simulink model "EKF"  (R2024b)
settings: Solver=FixedStepAuto  StartTime=0.0  StopTime=10  FixedStep=0.001  RelTol=1e-3
libraries: shared6dof x1, aerolibanim x1, simulink x1, aerolibnav x1
settings Model: Creator=cpero  LastModifiedBy=cpero

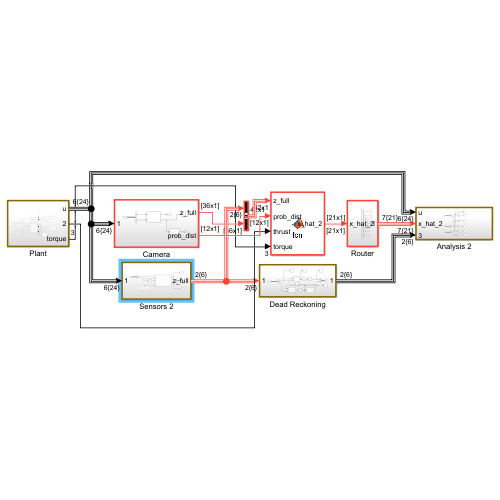
[thumbnail: Simulink's stored preview of the top-level diagram]
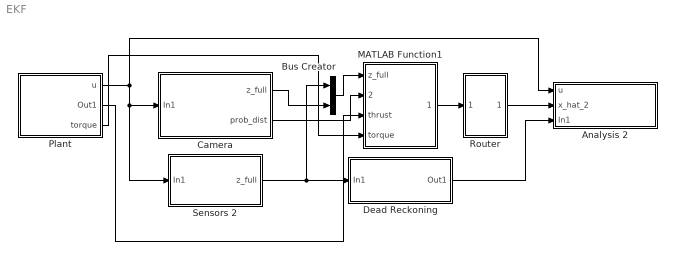
== system EKF ==
  Analysis 2 : Subsystem
  Bus Creator : BusCreator  Inputs=2
  Camera : Subsystem
  Dead Reckoning : Subsystem
  MATLAB Function1 : MATLAB Function  TreatAsAtomicUnit=on
  Plant : Subsystem
  Router : Subsystem
  Sensors 2 : Subsystem
  wires:
  Plant/1(u) -> Camera/1(In1), Sensors 2/1(In1), Analysis 2/1(u)
  Sensors 2/1(z_full) -> Bus Creator/1, Dead Reckoning/1(In1)
  Dead Reckoning/1(Out1) -> Analysis 2/3(In1)
  Router/1(Out1) -> Analysis 2/2(x_hat_2)
  MATLAB Function1/1(x_hat_2) -> Router/1(x_hat_2)
  Bus Creator/1 -> MATLAB Function1/1(z_full)
  Camera/1(z_full) -> Bus Creator/2
  Plant/2(Out1) -> MATLAB Function1/3(thrust)
  Camera/2(prob_dist) -> MATLAB Function1/2(prob_dist)
  Plant/3(torque) -> MATLAB Function1/4(torque)

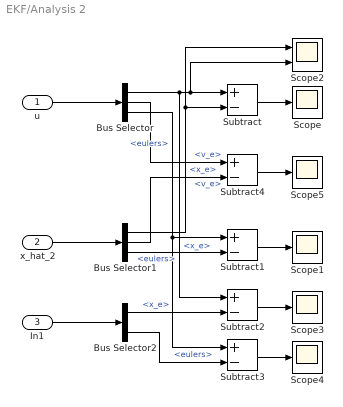
== system EKF/Analysis 2 ==
  u : Inport
  x_hat_2 : Inport  Port=2
  In1 : Inport  Port=3
  Bus Selector : BusSelector  OutputSignals=x_e,v_e,eulers
  Bus Selector1 : BusSelector  OutputSignals=x_e,v_e,eulers
  Bus Selector2 : BusSelector  OutputSignals=x_e,eulers
  Scope{,1,3..5} (5 alike) : Scope
  Scope2 : Scope  NumInputPorts=2
  Subtract{,1..4} (5 alike) : Sum  Inputs=+-
  wires:
  u/1 -> Bus Selector/1
  In1/1 -> Bus Selector2/1
  x_hat_2/1 -> Bus Selector1/1
  Bus Selector/1 -> Subtract2/1, Scope2/2, Subtract/1  "<x_e>"
  Bus Selector1/1 -> Scope2/1, Subtract/2  "<x_e>"
  Subtract/1 -> Scope/1
  Subtract1/1 -> Scope1/1
  Bus Selector/3 -> Subtract3/1, Subtract1/1  "<eulers>"
  Bus Selector1/3 -> Subtract1/2  "<eulers>"
  Subtract2/1 -> Scope3/1
  Bus Selector2/2 -> Subtract3/2  "<eulers>"
  Bus Selector2/1 -> Subtract2/2  "<x_e>"
  Subtract3/1 -> Scope4/1
  Subtract4/1 -> Scope5/1
  Bus Selector/2 -> Subtract4/1  "<v_e>"
  Bus Selector1/2 -> Subtract4/2  "<v_e>"

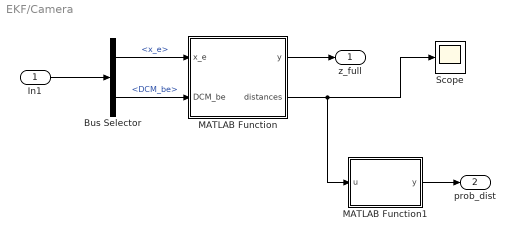
== system EKF/Camera ==
  In1 : Inport
  Bus Selector : BusSelector  OutputSignals=x_e,DCM_be
  MATLAB Function : MATLAB Function  TreatAsAtomicUnit=on
  MATLAB Function1 : MATLAB Function  TreatAsAtomicUnit=on
  Scope : Scope
  z_full : Outport
  prob_dist : Outport  Port=2
  wires:
  In1/1 -> Bus Selector/1
  Bus Selector/1 -> MATLAB Function/1(x_e)  "<x_e>"
  Bus Selector/2 -> MATLAB Function/2(DCM_be)  "<DCM_be>"
  MATLAB Function/1(y) -> z_full/1
  MATLAB Function/2(distances) -> MATLAB Function1/1(u), Scope/1
  MATLAB Function1/1(y) -> prob_dist/1

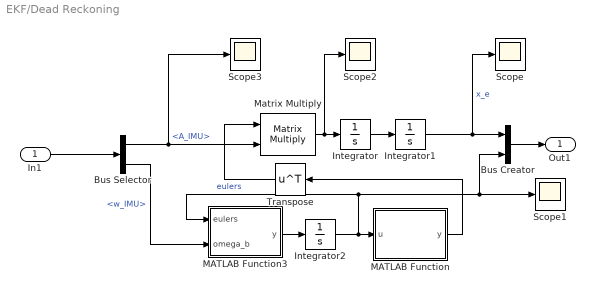
== system EKF/Dead Reckoning ==
  In1 : Inport
  Bus Creator : BusCreator  Inputs=2
  Bus Selector : BusSelector  OutputSignals=A_IMU,w_IMU
  Integrator : Integrator  InitialCondition=[0 0 1]
  Integrator1 : Integrator  InitialCondition=[0 0 1]
  Integrator2 : Integrator  InitialCondition=[0;0;0];
  MATLAB Function : MATLAB Function  TreatAsAtomicUnit=on
  MATLAB Function3 : MATLAB Function  TreatAsAtomicUnit=on
  Matrix Multiply : Product  Multiplication=Matrix(*)
  Scope{,1..3} (4 alike) : Scope
  Transpose : Math  Operator=transpose
  Out1 : Outport
  wires:
  Matrix Multiply/1 -> Scope2/1, Integrator/1
  Integrator/1 -> Integrator1/1
  In1/1 -> Bus Selector/1
  MATLAB Function3/1(y) -> Integrator2/1
  Integrator2/1 -> MATLAB Function/1(u), MATLAB Function3/1(eulers), Bus Creator/2, Scope1/1  "eulers"
  Integrator1/1 -> Scope/1, Bus Creator/1  "x_e"
  Bus Creator/1 -> Out1/1
  MATLAB Function/1(y) -> Transpose/1
  Transpose/1 -> Matrix Multiply/1
  Bus Selector/1 -> Scope3/1, Matrix Multiply/2  "<A_IMU>"
  Bus Selector/2 -> MATLAB Function3/2(omega_b)  "<w_IMU>"

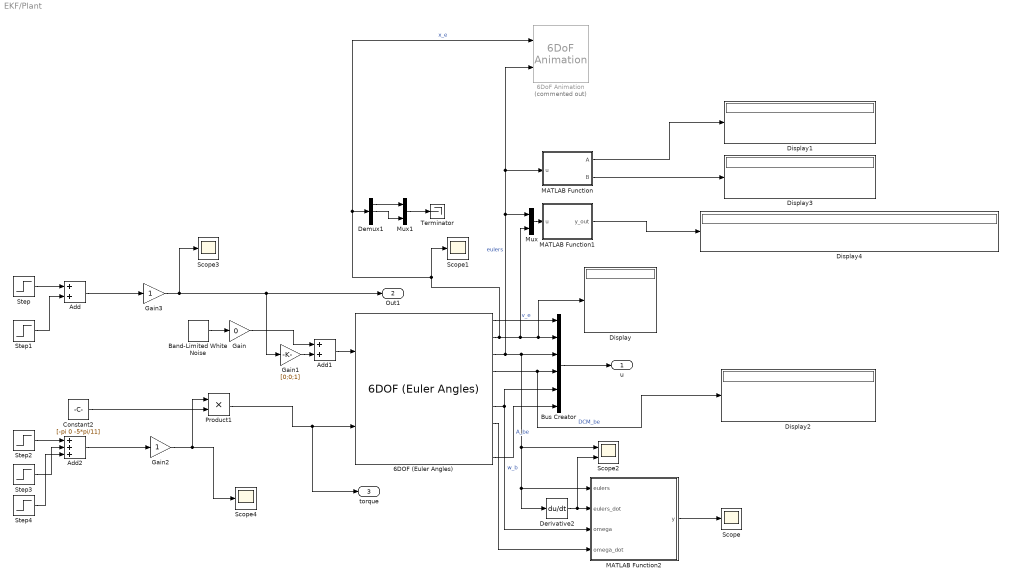
== system EKF/Plant ==
  6DOF (Euler Angles) : shared6dof/6DOF (Euler Angles)  units=Metric (MKS)  mtype=Fixed  rep=Euler Angles  xme_0=[0 0 1]  Vm_0=[0 0 1]  eul_0=[0 0 0]  pm_0=[0 0 0]  mass_0=1.0  mass_e=0.5  mass_f=2.0  inertia=eye(3)  inertia_e=eye(3)  inertia_f=2*eye(3)  k_quat=1.0  vre_flag=on  abi_flag=on  aMode=0  xme_statename=''  Vm_statename=''  eul_statename=''  quat_statename=''  pm_statename=''  mass_statename=''
  6DoF Animation : aerolibanim/6DoF Animation  Commented=on  u1=[-50 50 -50 50 0 50]  u2=0.1  u3=1.0  u4=[0 0 0]  u5=Cockpit  u6=[20 5 -31]  u7=10  u8=on
  Add : Sum
  Add1 : Sum
  Add2 : Sum  Inputs=+++
  Band-Limited White Noise : simulink/Sources/Band-Limited White Noise  Cov=[1e-5 1e-5 1e-5]  Ts=1e-3  seed=[76 34 60]
  Bus Creator : BusCreator  Inputs=6
  Constant2 : Constant  Value=[-pi 0 -5*pi/11]
  Demux1 : Demux  Outputs=3
  Derivative2 : Derivative
  Display{,1..4} (5 alike) : Display
  Gain : Gain  Gain=0
  Gain1 : Gain  Gain=[0;0;1]
  Gain2 : Gain
  Gain3 : Gain
  MATLAB Function : MATLAB Function  TreatAsAtomicUnit=on
  MATLAB Function1 : MATLAB Function  TreatAsAtomicUnit=on
  MATLAB Function2 : MATLAB Function  TreatAsAtomicUnit=on
  Mux : Mux  Inputs=2
  Mux1 : Mux  Inputs=2
  Product1 : Product
  Scope{,1,3..4} (4 alike) : Scope
  Scope2 : Scope  NumInputPorts=2
  Step : Step  SampleTime=0
  Step1 : Step  Time=2  After=-1  SampleTime=0
  Step2 : Step  Time=5  SampleTime=0
  Step3 : Step  Time=6  After=-2  SampleTime=0
  Step4 : Step  Time=7  SampleTime=0
  Terminator : Terminator
  u : Outport
  Out1 : Outport  Port=2
  torque : Outport  Port=3
  wires:
  6DOF (Euler Angles)/2 -> 6DoF Animation/1, Demux1/1, Scope1/1, Mux/2, Display/1, Bus Creator/2  "x_e"
  Bus Creator/1 -> u/1
  6DOF (Euler Angles)/4 -> Display2/1, Bus Creator/4  "DCM_be"
  6DOF (Euler Angles)/3 -> Mux/1, 6DoF Animation/2, MATLAB Function/1(u), MATLAB Function2/1(eulers), Derivative2/1, Scope2/1, Bus Creator/3  "eulers"
  6DOF (Euler Angles)/1 -> Bus Creator/1  "v_e"
  6DOF (Euler Angles)/9 -> Bus Creator/6  "A_be"
  6DOF (Euler Angles)/6 -> MATLAB Function2/3(omega), Bus Creator/5  "w_b"
  MATLAB Function/1(A) -> Display1/1
  MATLAB Function/2(B) -> Display3/1
  MATLAB Function1/1(y_out) -> Display4/1
  Mux/1 -> MATLAB Function1/1(u)
  6DOF (Euler Angles)/7 -> MATLAB Function2/4(omega_dot)
  Derivative2/1 -> Scope2/2, MATLAB Function2/2(eulers_dot)
  MATLAB Function2/1(y) -> Scope/1
  Constant2/1 -> Product1/2
  Demux1/2 -> Mux1/2
  Demux1/1 -> Mux1/1
  Mux1/1 -> Terminator/1
  Band-Limited White Noise/1 -> Gain/1
  Add1/1 -> 6DOF (Euler Angles)/1
  Gain/1 -> Add1/1
  Gain1/1 -> Add1/2
  Gain3/1 -> Scope3/1, Out1/1, Gain1/1
  Add2/1 -> Gain2/1
  Gain2/1 -> Scope4/1, Product1/1
  Step/1 -> Add/1
  Step1/1 -> Add/2
  Add/1 -> Gain3/1
  Step3/1 -> Add2/2
  Step2/1 -> Add2/1
  Step4/1 -> Add2/3
  Product1/1 -> torque/1, 6DOF (Euler Angles)/2

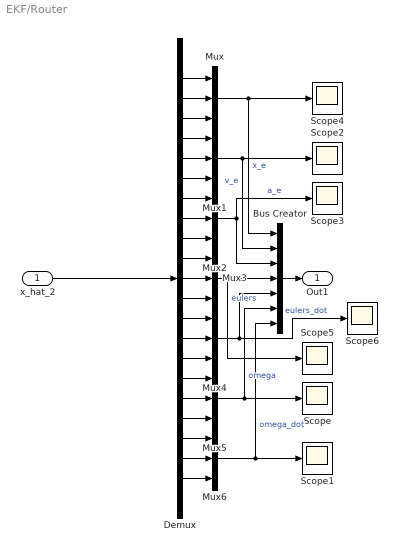
== system EKF/Router ==
  x_hat_2 : Inport
  Bus Creator : BusCreator  Inputs=7
  Demux : Demux  Outputs=21
  Mux{,1..6} (7 alike) : Mux  Inputs=3
  Scope{,1..6} (7 alike) : Scope
  Out1 : Outport
  wires:
  Demux/6 -> Mux1/3
  Mux2/1 -> Scope3/1, Bus Creator/3  "a_e"
  Demux/1 -> Mux/1
  Demux/15 -> Mux4/3
  Demux/18 -> Mux5/3
  Demux/12 -> Mux3/3
  Demux/13 -> Mux4/1
  Mux4/1 -> Scope6/1, Bus Creator/5  "eulers_dot"
  Demux/11 -> Mux3/2
  Mux5/1 -> Bus Creator/6, Scope/1  "omega"
  Demux/14 -> Mux4/2
  Demux/10 -> Mux3/1
  Mux1/1 -> Scope2/1, Bus Creator/2  "v_e"
  Demux/7 -> Mux2/1
  Demux/17 -> Mux5/2
  Demux/2 -> Mux/2
  Demux/5 -> Mux1/2
  Demux/4 -> Mux1/1
  Mux3/1 -> Scope5/1, Bus Creator/4  "eulers"
  Demux/3 -> Mux/3
  Demux/8 -> Mux2/2
  Demux/9 -> Mux2/3
  Demux/19 -> Mux6/1
  Mux/1 -> Scope4/1, Bus Creator/1  "x_e"
  Demux/16 -> Mux5/1
  Demux/20 -> Mux6/2
  Demux/21 -> Mux6/3
  Mux6/1 -> Bus Creator/7, Scope1/1  "omega_dot"
  x_hat_2/1 -> Demux/1
  Bus Creator/1 -> Out1/1

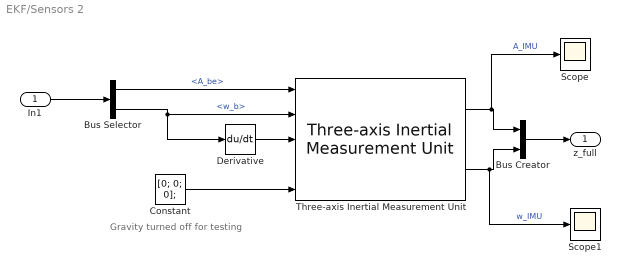
== system EKF/Sensors 2 ==
  note: Gravity turned off for testing
  In1 : Inport
  Bus Creator : BusCreator  Inputs=2
  Bus Selector : BusSelector  OutputSignals=A_be,w_b
  Constant : Constant  Value=[0; 0; 0];
  Derivative : Derivative
  Scope : Scope
  Scope1 : Scope
  Three-axis Inertial Measurement Unit : aerolibnav/Three-axis Inertial Measurement Unit  units=Metric (MKS)  imu=[0 0 0]  i_Ts=1e-3  dtype_a=off  w_a=190  z_a=0.707  a_sf_cc=[1 0 0; 0 1 0; 0 0 1]  a_bias=[0.02 -0.01 0.03]  a_sat="[-inf  -inf  -inf  inf inf inf]"  dtype_g=off  w_g=190  z_g=0.707  g_sf_cc=[1 0 0; 0 1 0; 0 0 1]  g_bias=[0.01 -0.02 0.03]  g_sens=[0 0 0]  g_sat="[-inf  -inf  -inf  inf inf inf]"  i_rand=on  i_seeds=[23093 23094 23095 23096 23097 23098]  i_pow=[1e-4 1e-4 1e-4 1e-6 1e-6 1e-6]
  z_full : Outport
  wires:
  In1/1 -> Bus Selector/1
  Bus Selector/1 -> Three-axis Inertial Measurement Unit/1  "<A_be>"
  Bus Selector/2 -> Derivative/1, Three-axis Inertial Measurement Unit/2  "<w_b>"
  Derivative/1 -> Three-axis Inertial Measurement Unit/3
  Constant/1 -> Three-axis Inertial Measurement Unit/5
  Three-axis Inertial Measurement Unit/1 -> Scope/1, Bus Creator/1  "A_IMU"
  Three-axis Inertial Measurement Unit/2 -> Scope1/1, Bus Creator/2  "w_IMU"
  Bus Creator/1 -> z_full/1

== matlab function EKF/Dead Reckoning/MATLAB Function3 ==
  data: eulers input; y output; omega_b input
function y = fcn(eulers, omega_b)

phi = eulers(1);
theta = eulers(2);
psi = eulers(3);

L = [1 sin(phi)*tan(theta) cos(phi)*tan(theta);
     0 cos(phi) -sin(phi);
     0 sin(phi)*sec(theta) cos(phi)*sec(theta)];

y = L*omega_b;

== matlab function EKF/Dead Reckoning/MATLAB Function ==
  data: u input; y output
function y = fcn(u)

y = angle2dcm(u(3),u(2),u(1));

phi = u(1);
theta = u(2);
psi = u(3);

B = [cos(psi)*cos(theta), cos(theta)*sin(psi), -sin(theta);
     cos(psi)*sin(theta)*sin(phi)-cos(phi)*sin(psi), cos(psi)*cos(phi)+sin(psi)*sin(theta)*sin(phi), cos(theta)*sin(phi);
     sin(psi)*sin(phi)+cos(psi)*cos(phi)*sin(theta), cos(phi)*sin(psi)*sin(theta)-cos(psi)*sin(phi), cos(theta)*cos(phi)];

== matlab function EKF/Plant/MATLAB Function ==
  data: u input; A output; B output
function [A, B] = fcn(u)

%phi
phi = u(1);
c = u(1);

theta = u(2);
b = u(2);

psi = u(3);
a = u(3);

%https://en.wikipedia.org/wiki/Euler_angles
%Transpose to go from DCM_eb to DCM_be
A = [cos(a)*cos(b), cos(a)*sin(b)*sin(c)-cos(c)*sin(a), sin(a)*sin(c)+cos(a)*cos(c)*sin(b);
     cos(b)*sin(a), cos(a)*cos(c)+sin(a)*sin(b)*sin(c), cos(c)*sin(a)*sin(b)-cos(a)*sin(c);
     -sin(b), cos(b)*sin(c), cos(b)*cos(c)]';

B = [cos(psi)*cos(theta), cos(theta)*sin(psi), -sin(theta);
     cos(psi)*sin(theta)*sin(phi)-cos(phi)*sin(psi), cos(psi)*cos(phi)+sin(psi)*sin(theta)*sin(phi), cos(theta)*sin(phi);
     sin(psi)*sin(phi)+cos(psi)*cos(phi)*sin(theta), cos(phi)*sin(psi)*sin(theta)-cos(psi)*sin(phi), cos(theta)*cos(phi)];

== matlab function EKF/Plant/MATLAB Function1 ==
  data: u input; y_out output
function y_out = fcn(u)

phi=u(1);
theta=u(2);
psi=u(3);
x=u(4);
y=u(5);
z=u(6);
a=-50;
b=120;
c=1;

y_out = reshape([0.0,1.0./sqrt((a-x).^2+(b-y).^2+(c-z).^2).*((sin(phi).*sin(psi)+cos(phi).*cos(psi).*sin(theta)).*(a-x)-(cos(psi).*sin(phi)-cos(phi).*sin(psi).*sin(theta)).*(b-y)+cos(phi).*cos(theta).*(c-z)),-1.0./sqrt((a-x).^2+(b-y).^2+(c-z).^2).*(-(cos(phi).*sin(psi)-cos(psi).*sin(phi).*sin(theta)).*(a-x)+(cos(phi).*cos(psi)+sin(phi).*sin(psi).*sin(theta)).*(b-y)+cos(theta).*sin(phi).*(c-z)),-1.0./sqrt((a-x).^2+(b-y).^2+(c-z).^2).*(cos(theta).*(c-z)+cos(psi).*sin(theta).*(a-x)+sin(psi).*sin(theta).*(b-y)),(-sin(phi).*sin(theta).*(c-z)+cos(psi).*cos(theta).*sin(phi).*(a-x)+cos(theta).*sin(phi).*sin(psi).*(b-y)).*1.0./sqrt((a-x).^2+(b-y).^2+(c-z).^2),(-cos(phi).*sin(theta).*(c-z)+cos(phi).*cos(psi).*cos(theta).*(a-x)+cos(phi).*cos(theta).*sin(psi).*(b-y)).*1.0./sqrt((a-x).^2+(b-y).^2+(c-z).^2),(cos(psi).*cos(theta).*(b-y)-cos(theta).*sin(psi).*(a-x)).*1.0./sqrt((a-x).^2+(b-y).^2+(c-z).^2),-((cos(phi).*cos(psi)+sin(phi).*sin(psi).*sin(theta)).*(a-x)+(cos(phi).*sin(psi)-cos(psi).*sin(phi).*sin(theta)).*(b-y)).*1.0./sqrt((a-x).^2+(b-y).^2+(c-z).^2),((cos(psi).*sin(phi)-cos(phi).*sin(psi).*sin(theta)).*(a-x)+(sin(phi).*sin(psi)+cos(phi).*cos(psi).*sin(theta)).*(b-y)).*1.0./sqrt((a-x).^2+(b-y).^2+(c-z).^2),((a.*2.0-x.*2.0).*1.0./((a-x).^2+(b-y).^2+(c-z).^2).^(3.0./2.0).*(-sin(theta).*(c-z)+cos(psi).*cos(theta).*(a-x)+cos(theta).*sin(psi).*(b-y)))./2.0-cos(psi).*cos(theta).*1.0./sqrt((a-x).^2+(b-y).^2+(c-z).^2),(cos(phi).*sin(psi)-cos(psi).*sin(phi).*sin(theta)).*1.0./sqrt((a-x).^2+(b-y).^2+(c-z).^2)+((a.*2.0-x.*2.0).*1.0./((a-x).^2+(b-y).^2+(c-z).^2).^(3.0./2.0).*(-(cos(phi).*sin(psi)-cos(psi).*sin(phi).*sin(theta)).*(a-x)+(cos(phi).*cos(psi)+sin(phi).*sin(psi).*sin(theta)).*(b-y)+cos(theta).*sin(phi).*(c-z)))./2.0,-(sin(phi).*sin(psi)+cos(phi).*cos(psi).*sin(theta)).*1.0./sqrt((a-x).^2+(b-y).^2+(c-z).^2)+((a.*2.0-x.*2.0).*1.0./((a-x).^2+(b-y).^2+(c-z).^2).^(3.0./2.0).*((sin(phi).*sin(psi)+cos(phi).*cos(psi).*sin(theta)).*(a-x)-(cos(psi).*sin(phi)-cos(phi).*sin(psi).*sin(theta)).*(b-y)+cos(phi).*cos(theta).*(c-z)))./2.0,((b.*2.0-y.*2.0).*1.0./((a-x).^2+(b-y).^2+(c-z).^2).^(3.0./2.0).*(-sin(theta).*(c-z)+cos(psi).*cos(theta).*(a-x)+cos(theta).*sin(psi).*(b-y)))./2.0-cos(theta).*sin(psi).*1.0./sqrt((a-x).^2+(b-y).^2+(c-z).^2),-(cos(phi).*cos(psi)+sin(phi).*sin(psi).*sin(theta)).*1.0./sqrt((a-x).^2+(b-y).^2+(c-z).^2)+((b.*2.0-y.*2.0).*1.0./((a-x).^2+(b-y).^2+(c-z).^2).^(3.0./2.0).*(-(cos(phi).*sin(psi)-cos(psi).*sin(phi).*sin(theta)).*(a-x)+(cos(phi).*cos(psi)+sin(phi).*sin(psi).*sin(theta)).*(b-y)+cos(theta).*sin(phi).*(c-z)))./2.0,(cos(psi).*sin(phi)-cos(phi).*sin(psi).*sin(theta)).*1.0./sqrt((a-x).^2+(b-y).^2+(c-z).^2)+((b.*2.0-y.*2.0).*1.0./((a-x).^2+(b-y).^2+(c-z).^2).^(3.0./2.0).*((sin(phi).*sin(psi)+cos(phi).*cos(psi).*sin(theta)).*(a-x)-(cos(psi).*sin(phi)-cos(phi).*sin(psi).*sin(theta)).*(b-y)+cos(phi).*cos(theta).*(c-z)))./2.0,sin(theta).*1.0./sqrt((a-x).^2+(b-y).^2+(c-z).^2)+((c.*2.0-z.*2.0).*1.0./((a-x).^2+(b-y).^2+(c-z).^2).^(3.0./2.0).*(-sin(theta).*(c-z)+cos(psi).*cos(theta).*(a-x)+cos(theta).*sin(psi).*(b-y)))./2.0,-cos(theta).*sin(phi).*1.0./sqrt((a-x).^2+(b-y).^2+(c-z).^2)+((c.*2.0-z.*2.0).*1.0./((a-x).^2+(b-y).^2+(c-z).^2).^(3.0./2.0).*(-(cos(phi).*sin(psi)-cos(psi).*sin(phi).*sin(theta)).*(a-x)+(cos(phi).*cos(psi)+sin(phi).*sin(psi).*sin(theta)).*(b-y)+cos(theta).*sin(phi).*(c-z)))./2.0,-cos(phi).*cos(theta).*1.0./sqrt((a-x).^2+(b-y).^2+(c-z).^2)+((c.*2.0-z.*2.0).*1.0./((a-x).^2+(b-y).^2+(c-z).^2).^(3.0./2.0).*((sin(phi).*sin(psi)+cos(phi).*cos(psi).*sin(theta)).*(a-x)-(cos(psi).*sin(phi)-cos(phi).*sin(psi).*sin(theta)).*(b-y)+cos(phi).*cos(theta).*(c-z)))./2.0],[3,6]);

== matlab function EKF/Plant/MATLAB Function2 ==
  data: eulers input; eulers_dot input; omega input; y output; omega_dot input
function y = fcn(eulers, eulers_dot, omega, omega_dot)

phi = eulers(1);
theta = eulers(2);
psi = eulers(3);
phi_dot = eulers_dot(1);
theta_dot = eulers_dot(2);
psi_dot = eulers_dot(3);

L = [1 sin(phi)*tan(theta) cos(phi)*tan(theta);
     0 cos(phi) -sin(phi);
     0 sin(phi)*sec(theta) cos(phi)*sec(theta)];

L_prime = [0, sin(phi)*(sec(theta)^2)*theta_dot + tan(theta)*cos(phi)*phi_dot, cos(phi)*(sec(theta)^2)*theta_dot - tan(theta)*sin(phi)*phi_dot;
           0, -sin(phi)*phi_dot, -cos(phi)*phi_dot;
           0, sin(phi)*(tan(theta)*sec(theta))*theta_dot + sec(theta)*cos(phi)*phi_dot, cos(phi)*(tan(theta)*sec(theta))*theta_dot - sec(theta)*sin(phi)*phi_dot];

y = (L*omega_dot) + (L_prime*omega);

== matlab function EKF/Camera/MATLAB Function ==
  settings: updateMethod=DISCRETE
  data: x_e input; y output; DCM_be input; marker_data parameter; distances output
function [y, distances] = fcn(x_e, DCM_be, marker_data)
N = size(marker_data, 2);

distances = zeros(N,1);
y = zeros(N*3,1);
for i=1:N
    delta = DCM_be*(marker_data(:,i) - x_e);
    rho = delta/(norm(delta));
    distances(i) = norm(delta); 
    y(1+(3*(i-1)):3+(3*(i-1))) = rho + normrnd(0,1e-2,[3,1]);
end

== matlab function EKF/MATLAB Function1 ==
  settings: updateMethod=DISCRETE
  data: z_full input; prob_dist input; x_hat_2 output; marker_data parameter; thrust input; torque input
function x_hat_2  = fcn(z_full, prob_dist, marker_data, thrust, torque)

persistent x_hat_2_prior P_hat_2_prior j

if isempty(x_hat_2_prior)
    x_hat_2_prior = zeros(21,1);
    x_hat_2_prior(1:3) = [0 0 1];
    x_hat_2_prior(4:6) = [0 0 1];
    x_hat_2_prior(7:9) = [0 0 0];
    P_hat_2_prior = kron(diag([1e-4 1e-4 1e-4 1e-4 1e-6 1e-6 1e-6]),eye(3));
    x_hat_2_prior(10:12) = [0 0 0];
    x_hat_2_prior(13:15) = [0 0 0];
    x_hat_2_prior(16:18) = [0 0 0];
    j=0;
end

rho_num = size(marker_data, 2);

accel_vec = ones(1,3);
gyro_vec = ones(1,3);
rho_vec = zeros(1,3*rho_num);

rho_calc_required = false;
if true
    rng(j);
    num_tries=5;
    random_rhos = randi(rho_num,[1,num_tries]);
    for k=1:num_tries
        cdf = cumsum(prob_dist);
        random_value = rand();
        random_rho = find(random_value <= cdf, 1);
        rho_vec(3*(random_rho(1)-1)+1:3*random_rho(1)) = ones(1,3);
    end
    sensor_vec = [accel_vec, gyro_vec, rho_vec];
    rho_calc_required = true;
else
    sensor_vec = [accel_vec, gyro_vec, zeros(1,3*rho_num)];
end

j = j+1;

dt = 1e-3;

Q = kron(diag([0 0 0 0 0 0 0]),eye(3));
rho_R_vec = 1e-2*ones(1,rho_num);
R_full = kron(diag([1e-1 1e-1 rho_R_vec]),eye(3));

[r1, r2, r3] = deal(x_hat_2_prior(1), x_hat_2_prior(2), x_hat_2_prior(3));
[r_dot1, r_dot2, r_dot3] = deal(x_hat_2_prior(4), x_hat_2_prior(5), x_hat_2_prior(6));
[r_dot_dot1, r_dot_dot2, r_dot_dot3] = deal(x_hat_2_prior(7), x_hat_2_prior(8), x_hat_2_prior(9));
[eulers1, eulers2, eulers3] = deal(x_hat_2_prior(10), x_hat_2_prior(11), x_hat_2_prior(12));
[eulers_dot1, eulers_dot2, eulers_dot3] = deal(x_hat_2_prior(13), x_hat_2_prior(14), x_hat_2_prior(15));
[omega1, omega2, omega3] = deal(x_hat_2_prior(16), x_hat_2_prior(17), x_hat_2_prior(18));
[omega_dot1, omega_dot2, omega_dot3] = deal(x_hat_2_prior(19), x_hat_2_prior(20), x_hat_2_prior(21));

torque1 = torque(1); 
torque2 = torque(2);
torque3 = torque(3);
mass = 1;

%Predict
x_hat_1 = [r1+dt.*r_dot1+(dt.^2.*r_dot_dot1)./2.0;r2+dt.*r_dot2+(dt.^2.*r_dot_dot2)./2.0;r3+dt.*r_dot3+(dt.^2.*r_dot_dot3)./2.0;r_dot1+dt.*r_dot_dot1;r_dot2+dt.*r_dot_dot2;r_dot3+dt.*r_dot_dot3;(thrust.*(sin(eulers1).*sin(eulers3)+cos(eulers1).*cos(eulers3).*sin(eulers2)))./mass;-(thrust.*(cos(eulers3).*sin(eulers1)-cos(eulers1).*sin(eulers2).*sin(eulers3)))./mass;(thrust.*cos(eulers1).*cos(eulers2))./mass;eulers1+dt.*eulers_dot1;eulers2+dt.*eulers_dot2;eulers3+dt.*eulers_dot3;eulers_dot1+dt.*(omega_dot1+omega2.*(eulers_dot1.*cos(eulers1).*tan(eulers2)+eulers_dot2.*1.0./cos(eulers2).^2.*sin(eulers1))-omega3.*(eulers_dot1.*sin(eulers1).*tan(eulers2)-eulers_dot2.*cos(eulers1).*1.0./cos(eulers2).^2)+omega_dot3.*cos(eulers1).*tan(eulers2)+omega_dot2.*sin(eulers1).*tan(eulers2));eulers_dot2-dt.*(-omega_dot2.*cos(eulers1)+omega_dot3.*sin(eulers1)+eulers_dot1.*omega2.*sin(eulers1)+eulers_dot1.*omega3.*cos(eulers1));eulers_dot3+dt.*(omega2.*((eulers_dot1.*cos(eulers1))./cos(eulers2)+(eulers_dot2.*sin(eulers1).*tan(eulers2))./cos(eulers2))-omega3.*((eulers_dot1.*sin(eulers1))./cos(eulers2)-(eulers_dot2.*cos(eulers1).*tan(eulers2))./cos(eulers2))+(omega_dot3.*cos(eulers1))./cos(eulers2)+(omega_dot2.*sin(eulers1))./cos(eulers2));omega1+dt.*omega_dot1;omega2+dt.*omega_dot2;omega3+dt.*omega_dot3;torque1;torque2;torque3];
F_jacobian = reshape([1.0,0.0,0.0,0.0,0.0,0.0,0.0,0.0,0.0,0.0,0.0,0.0,0.0,0.0,0.0,0.0,0.0,0.0,0.0,0.0,0.0,0.0,1.0,0.0,0.0,0.0,0.0,0.0,0.0,0.0,0.0,0.0,0.0,0.0,0.0,0.0,0.0,0.0,0.0,0.0,0.0,0.0,0.0,0.0,1.0,0.0,0.0,0.0,0.0,0.0,0.0,0.0,0.0,0.0,0.0,0.0,0.0,0.0,0.0,0.0,0.0,0.0,0.0,dt,0.0,0.0,1.0,0.0,0.0,0.0,0.0,0.0,0.0,0.0,0.0,0.0,0.0,0.0,0.0,0.0,0.0,0.0,0.0,0.0,0.0,dt,0.0,0.0,1.0,0.0,0.0,0.0,0.0,0.0,0.0,0.0,0.0,0.0,0.0,0.0,0.0,0.0,0.0,0.0,0.0,0.0,0.0,dt,0.0,0.0,1.0,0.0,0.0,0.0,0.0,0.0,0.0,0.0,0.0,0.0,0.0,0.0,0.0,0.0,0.0,0.0,dt.^2./2.0,0.0,0.0,dt,0.0,0.0,0.0,0.0,0.0,0.0,0.0,0.0,0.0,0.0,0.0,0.0,0.0,0.0,0.0,0.0,0.0,0.0,dt.^2./2.0,0.0,0.0,dt,0.0,0.0,0.0,0.0,0.0,0.0,0.0,0.0,0.0,0.0,0.0,0.0,0.0,0.0,0.0,0.0,0.0,0.0,dt.^2./2.0,0.0,0.0,dt,0.0,0.0,0.0,0.0,0.0,0.0,0.0,0.0,0.0,0.0,0.0,0.0,0.0,0.0,0.0,0.0,0.0,0.0,0.0,0.0,0.0,(thrust.*(cos(eulers1).*sin(eulers3)-cos(eulers3).*sin(eulers1).*sin(eulers2)))./mass,-(thrust.*(cos(eulers1).*cos(eulers3)+sin(eulers1).*sin(eulers2).*sin(eulers3)))./mass,-(thrust.*cos(eulers2).*sin(eulers1))./mass,1.0,0.0,0.0,-dt.*(omega2.*(eulers_dot1.*sin(eulers1).*tan(eulers2)-eulers_dot2.*cos(eulers1).*1.0./cos(eulers2).^2)+omega3.*(eulers_dot1.*cos(eulers1).*tan(eulers2)+eulers_dot2.*1.0./cos(eulers2).^2.*sin(eulers1))-omega_dot2.*cos(eulers1).*tan(eulers2)+omega_dot3.*sin(eulers1).*tan(eulers2)),-dt.*(omega_dot3.*cos(eulers1)+omega_dot2.*sin(eulers1)-eulers_dot1.*omega3.*sin(eulers1)+eulers_dot1.*omega2.*cos(eulers1)),-dt.*(omega2.*((eulers_dot1.*sin(eulers1))./cos(eulers2)-(eulers_dot2.*cos(eulers1).*tan(eulers2))./cos(eulers2))+omega3.*((eulers_dot1.*cos(eulers1))./cos(eulers2)+(eulers_dot2.*sin(eulers1).*tan(eulers2))./cos(eulers2))-(omega_dot2.*cos(eulers1))./cos(eulers2)+(omega_dot3.*sin(eulers1))./cos(eulers2)),0.0,0.0,0.0,0.0,0.0,0.0,0.0,0.0,0.0,0.0,0.0,0.0,(thrust.*cos(eulers1).*cos(eulers2).*cos(eulers3))./mass,(thrust.*cos(eulers1).*cos(eulers2).*sin(eulers3))./mass,-(thrust.*cos(eulers1).*sin(eulers2))./mass,0.0,1.0,0.0,dt.*(omega2.*(eulers_dot1.*cos(eulers1).*(tan(eulers2).^2+1.0)+eulers_dot2.*1.0./cos(eulers2).^3.*sin(eulers1).*sin(eulers2).*2.0)-omega3.*(eulers_dot1.*sin(eulers1).*(tan(eulers2).^2+1.0)-eulers_dot2.*cos(eulers1).*1.0./cos(eulers2).^3.*sin(eulers2).*2.0)+omega_dot3.*cos(eulers1).*(tan(eulers2).^2+1.0)+omega_dot2.*sin(eulers1).*(tan(eulers2).^2+1.0)),0.0,dt.*(omega3.*((eulers_dot2.*cos(eulers1).*(tan(eulers2).^2+1.0))./cos(eulers2)-eulers_dot1.*1.0./cos(eulers2).^2.*sin(eulers1).*sin(eulers2)+eulers_dot2.*cos(eulers1).*1.0./cos(eulers2).^2.*sin(eulers2).*tan(eulers2))+omega2.*((eulers_dot2.*sin(eulers1).*(tan(eulers2).^2+1.0))./cos(eulers2)+eulers_dot1.*cos(eulers1).*1.0./cos(eulers2).^2.*sin(eulers2)+eulers_dot2.*1.0./cos(eulers2).^2.*sin(eulers1).*sin(eulers2).*tan(eulers2))+omega_dot3.*cos(eulers1).*1.0./cos(eulers2).^2.*sin(eulers2)+omega_dot2.*1.0./cos(eulers2).^2.*sin(eulers1).*sin(eulers2)),0.0,0.0,0.0,0.0,0.0,0.0,0.0,0.0,0.0,0.0,0.0,0.0,(thrust.*(cos(eulers3).*sin(eulers1)-cos(eulers1).*sin(eulers2).*sin(eulers3)))./mass,(thrust.*(sin(eulers1).*sin(eulers3)+cos(eulers1).*cos(eulers3).*sin(eulers2)))./mass,0.0,0.0,0.0,1.0,0.0,0.0,0.0,0.0,0.0,0.0,0.0,0.0,0.0,0.0,0.0,0.0,0.0,0.0,0.0,0.0,0.0,0.0,dt,0.0,0.0,dt.*(omega2.*cos(eulers1).*tan(eulers2)-omega3.*sin(eulers1).*tan(eulers2))+1.0,-dt.*(omega3.*cos(eulers1)+omega2.*sin(eulers1)),dt.*((omega2.*cos(eulers1))./cos(eulers2)-(omega3.*sin(eulers1))./cos(eulers2)),0.0,0.0,0.0,0.0,0.0,0.0,0.0,0.0,0.0,0.0,0.0,0.0,0.0,0.0,0.0,0.0,dt,0.0,dt.*(omega3.*cos(eulers1).*1.0./cos(eulers2).^2+omega2.*1.0./cos(eulers2).^2.*sin(eulers1)),1.0,dt.*((omega3.*cos(eulers1).*tan(eulers2))./cos(eulers2)+(omega2.*sin(eulers1).*tan(eulers2))./cos(eulers2)),0.0,0.0,0.0,0.0,0.0,0.0,0.0,0.0,0.0,0.0,0.0,0.0,0.0,0.0,0.0,0.0,0.0,dt,0.0,0.0,1.0,0.0,0.0,0.0,0.0,0.0,0.0,0.0,0.0,0.0,0.0,0.0,0.0,0.0,0.0,0.0,0.0,0.0,0.0,0.0,0.0,0.0,1.0,0.0,0.0,0.0,0.0,0.0,0.0,0.0,0.0,0.0,0.0,0.0,0.0,0.0,0.0,0.0,0.0,0.0,dt.*(eulers_dot1.*cos(eulers1).*tan(eulers2)+eulers_dot2.*1.0./cos(eulers2).^2.*sin(eulers1)),-dt.*eulers_dot1.*sin(eulers1),dt.*((eulers_dot1.*cos(eulers1))./cos(eulers2)+(eulers_dot2.*sin(eulers1).*tan(eulers2))./cos(eulers2)),0.0,1.0,0.0,0.0,0.0,0.0,0.0,0.0,0.0,0.0,0.0,0.0,0.0,0.0,0.0,0.0,0.0,0.0,-dt.*(eulers_dot1.*sin(eulers1).*tan(eulers2)-eulers_dot2.*cos(eulers1).*1.0./cos(eulers2).^2),-dt.*eulers_dot1.*cos(eulers1),-dt.*((eulers_dot1.*sin(eulers1))./cos(eulers2)-(eulers_dot2.*cos(eulers1).*tan(eulers2))./cos(eulers2)),0.0,0.0,1.0,0.0,0.0,0.0,0.0,0.0,0.0,0.0,0.0,0.0,0.0,0.0,0.0,0.0,0.0,0.0,dt,0.0,0.0,dt,0.0,0.0,0.0,0.0,0.0,0.0,0.0,0.0,0.0,0.0,0.0,0.0,0.0,0.0,0.0,0.0,0.0,dt.*sin(eulers1).*tan(eulers2),dt.*cos(eulers1),(dt.*sin(eulers1))./cos(eulers2),0.0,dt,0.0,0.0,0.0,0.0,0.0,0.0,0.0,0.0,0.0,0.0,0.0,0.0,0.0,0.0,0.0,0.0,dt.*cos(eulers1).*tan(eulers2),-dt.*sin(eulers1),(dt.*cos(eulers1))./cos(eulers2),0.0,0.0,dt,0.0,0.0,0.0],[21,21]);
P_hat_1 = F_jacobian*P_hat_2_prior*F_jacobian' + Q;

%Update
num_states = 21;

rho_prediction = zeros(rho_num*3,1);
H_jacobian_rho = zeros(rho_num*3,21);
if rho_calc_required
    for i=1:rho_num
        marker1 = marker_data(1,i);
        marker2 = marker_data(2,i);
        marker3 = marker_data(3,i);
        rho_prediction(1+(3*(i-1)):3+(3*(i-1))) = [1.0./sqrt((marker1-r1).^2+(marker2-r2).^2+(marker3-r3).^2).*(-sin(eulers2).*(marker3-r3)+cos(eulers2).*cos(eulers3).*(marker1-r1)+cos(eulers2).*sin(eulers3).*(marker2-r2));
            1.0./sqrt((marker1-r1).^2+(marker2-r2).^2+(marker3-r3).^2).*(-(cos(eulers1).*sin(eulers3)-cos(eulers3).*sin(eulers1).*sin(eulers2)).*(marker1-r1)+(cos(eulers1).*cos(eulers3)+sin(eulers1).*sin(eulers2).*sin(eulers3)).*(marker2-r2)+cos(eulers2).*sin(eulers1).*(marker3-r3));
            1.0./sqrt((marker1-r1).^2+(marker2-r2).^2+(marker3-r3).^2).*((sin(eulers1).*sin(eulers3)+cos(eulers1).*cos(eulers3).*sin(eulers2)).*(marker1-r1)-(cos(eulers3).*sin(eulers1)-cos(eulers1).*sin(eulers2).*sin(eulers3)).*(marker2-r2)+cos(eulers1).*cos(eulers2).*(marker3-r3))];
        H_jacobian_rho(1+(3*(i-1)):3+(3*(i-1)),:) = reshape([((marker1.*2.0-r1.*2.0).*1.0./((marker1-r1).^2+(marker2-r2).^2+(marker3-r3).^2).^(3.0./2.0).*(-sin(eulers2).*(marker3-r3)+cos(eulers2).*cos(eulers3).*(marker1-r1)+cos(eulers2).*sin(eulers3).*(marker2-r2)))./2.0-cos(eulers2).*cos(eulers3).*1.0./sqrt((marker1-r1).^2+(marker2-r2).^2+(marker3-r3).^2),(cos(eulers1).*sin(eulers3)-cos(eulers3).*sin(eulers1).*sin(eulers2)).*1.0./sqrt((marker1-r1).^2+(marker2-r2).^2+(marker3-r3).^2)+((marker1.*2.0-r1.*2.0).*1.0./((marker1-r1).^2+(marker2-r2).^2+(marker3-r3).^2).^(3.0./2.0).*(-(cos(eulers1).*sin(eulers3)-cos(eulers3).*sin(eulers1).*sin(eulers2)).*(marker1-r1)+(cos(eulers1).*cos(eulers3)+sin(eulers1).*sin(eulers2).*sin(eulers3)).*(marker2-r2)+cos(eulers2).*sin(eulers1).*(marker3-r3)))./2.0,-(sin(eulers1).*sin(eulers3)+cos(eulers1).*cos(eulers3).*sin(eulers2)).*1.0./sqrt((marker1-r1).^2+(marker2-r2).^2+(marker3-r3).^2)+((marker1.*2.0-r1.*2.0).*1.0./((marker1-r1).^2+(marker2-r2).^2+(marker3-r3).^2).^(3.0./2.0).*((sin(eulers1).*sin(eulers3)+cos(eulers1).*cos(eulers3).*sin(eulers2)).*(marker1-r1)-(cos(eulers3).*sin(eulers1)-cos(eulers1).*sin(eulers2).*sin(eulers3)).*(marker2-r2)+cos(eulers1).*cos(eulers2).*(marker3-r3)))./2.0,((marker2.*2.0-r2.*2.0).*1.0./((marker1-r1).^2+(marker2-r2).^2+(marker3-r3).^2).^(3.0./2.0).*(-sin(eulers2).*(marker3-r3)+cos(eulers2).*cos(eulers3).*(marker1-r1)+cos(eulers2).*sin(eulers3).*(marker2-r2)))./2.0-cos(eulers2).*sin(eulers3).*1.0./sqrt((marker1-r1).^2+(marker2-r2).^2+(marker3-r3).^2),-(cos(eulers1).*cos(eulers3)+sin(eulers1).*sin(eulers2).*sin(eulers3)).*1.0./sqrt((marker1-r1).^2+(marker2-r2).^2+(marker3-r3).^2)+((marker2.*2.0-r2.*2.0).*1.0./((marker1-r1).^2+(marker2-r2).^2+(marker3-r3).^2).^(3.0./2.0).*(-(cos(eulers1).*sin(eulers3)-cos(eulers3).*sin(eulers1).*sin(eulers2)).*(marker1-r1)+(cos(eulers1).*cos(eulers3)+sin(eulers1).*sin(eulers2).*sin(eulers3)).*(marker2-r2)+cos(eulers2).*sin(eulers1).*(marker3-r3)))./2.0,(cos(eulers3).*sin(eulers1)-cos(eulers1).*sin(eulers2).*sin(eulers3)).*1.0./sqrt((marker1-r1).^2+(marker2-r2).^2+(marker3-r3).^2)+((marker2.*2.0-r2.*2.0).*1.0./((marker1-r1).^2+(marker2-r2).^2+(marker3-r3).^2).^(3.0./2.0).*((sin(eulers1).*sin(eulers3)+cos(eulers1).*cos(eulers3).*sin(eulers2)).*(marker1-r1)-(cos(eulers3).*sin(eulers1)-cos(eulers1).*sin(eulers2).*sin(eulers3)).*(marker2-r2)+cos(eulers1).*cos(eulers2).*(marker3-r3)))./2.0,sin(eulers2).*1.0./sqrt((marker1-r1).^2+(marker2-r2).^2+(marker3-r3).^2)+((marker3.*2.0-r3.*2.0).*1.0./((marker1-r1).^2+(marker2-r2).^2+(marker3-r3).^2).^(3.0./2.0).*(-sin(eulers2).*(marker3-r3)+cos(eulers2).*cos(eulers3).*(marker1-r1)+cos(eulers2).*sin(eulers3).*(marker2-r2)))./2.0,((marker3.*2.0-r3.*2.0).*1.0./((marker1-r1).^2+(marker2-r2).^2+(marker3-r3).^2).^(3.0./2.0).*(-(cos(eulers1).*sin(eulers3)-cos(eulers3).*sin(eulers1).*sin(eulers2)).*(marker1-r1)+(cos(eulers1).*cos(eulers3)+sin(eulers1).*sin(eulers2).*sin(eulers3)).*(marker2-r2)+cos(eulers2).*sin(eulers1).*(marker3-r3)))./2.0-cos(eulers2).*sin(eulers1).*1.0./sqrt((marker1-r1).^2+(marker2-r2).^2+(marker3-r3).^2),((marker3.*2.0-r3.*2.0).*1.0./((marker1-r1).^2+(marker2-r2).^2+(marker3-r3).^2).^(3.0./2.0).*((sin(eulers1).*sin(eulers3)+cos(eulers1).*cos(eulers3).*sin(eulers2)).*(marker1-r1)-(cos(eulers3).*sin(eulers1)-cos(eulers1).*sin(eulers2).*sin(eulers3)).*(marker2-r2)+cos(eulers1).*cos(eulers2).*(marker3-r3)))./2.0-cos(eulers1).*cos(eulers2).*1.0./sqrt((marker1-r1).^2+(marker2-r2).^2+(marker3-r3).^2),0.0,0.0,0.0,0.0,0.0,0.0,0.0,0.0,0.0,0.0,0.0,0.0,0.0,0.0,0.0,0.0,0.0,0.0,0.0,1.0./sqrt((marker1-r1).^2+(marker2-r2).^2+(marker3-r3).^2).*((sin(eulers1).*sin(eulers3)+cos(eulers1).*cos(eulers3).*sin(eulers2)).*(marker1-r1)-(cos(eulers3).*sin(eulers1)-cos(eulers1).*sin(eulers2).*sin(eulers3)).*(marker2-r2)+cos(eulers1).*cos(eulers2).*(marker3-r3)),-1.0./sqrt((marker1-r1).^2+(marker2-r2).^2+(marker3-r3).^2).*(-(cos(eulers1).*sin(eulers3)-cos(eulers3).*sin(eulers1).*sin(eulers2)).*(marker1-r1)+(cos(eulers1).*cos(eulers3)+sin(eulers1).*sin(eulers2).*sin(eulers3)).*(marker2-r2)+cos(eulers2).*sin(eulers1).*(marker3-r3)),-1.0./sqrt((marker1-r1).^2+(marker2-r2).^2+(marker3-r3).^2).*(cos(eulers2).*(marker3-r3)+cos(eulers3).*sin(eulers2).*(marker1-r1)+sin(eulers2).*sin(eulers3).*(marker2-r2)),1.0./sqrt((marker1-r1).^2+(marker2-r2).^2+(marker3-r3).^2).*(-sin(eulers1).*sin(eulers2).*(marker3-r3)+cos(eulers2).*cos(eulers3).*sin(eulers1).*(marker1-r1)+cos(eulers2).*sin(eulers1).*sin(eulers3).*(marker2-r2)),1.0./sqrt((marker1-r1).^2+(marker2-r2).^2+(marker3-r3).^2).*(-cos(eulers1).*sin(eulers2).*(marker3-r3)+cos(eulers1).*cos(eulers2).*cos(eulers3).*(marker1-r1)+cos(eulers1).*cos(eulers2).*sin(eulers3).*(marker2-r2)),(cos(eulers2).*cos(eulers3).*(marker2-r2)-cos(eulers2).*sin(eulers3).*(marker1-r1)).*1.0./sqrt((marker1-r1).^2+(marker2-r2).^2+(marker3-r3).^2),-((cos(eulers1).*cos(eulers3)+sin(eulers1).*sin(eulers2).*sin(eulers3)).*(marker1-r1)+(cos(eulers1).*sin(eulers3)-cos(eulers3).*sin(eulers1).*sin(eulers2)).*(marker2-r2)).*1.0./sqrt((marker1-r1).^2+(marker2-r2).^2+(marker3-r3).^2),((cos(eulers3).*sin(eulers1)-cos(eulers1).*sin(eulers2).*sin(eulers3)).*(marker1-r1)+(sin(eulers1).*sin(eulers3)+cos(eulers1).*cos(eulers3).*sin(eulers2)).*(marker2-r2)).*1.0./sqrt((marker1-r1).^2+(marker2-r2).^2+(marker3-r3).^2),0.0,0.0,0.0,0.0,0.0,0.0,0.0,0.0,0.0,0.0,0.0,0.0,0.0,0.0,0.0,0.0,0.0,0.0,0.0,0.0,0.0,0.0,0.0,0.0,0.0,0.0,0.0],[3,21]);
        i = i+1;
    end
end

omega_prediction = [omega1; omega2; omega3];
accel_prediction = [r_dot_dot1; r_dot_dot2; r_dot_dot3];

H_jacobian_accel = reshape([0.0,0.0,0.0,0.0,0.0,0.0,0.0,0.0,0.0,0.0,0.0,0.0,0.0,0.0,0.0,0.0,0.0,0.0,cos(eulers2).*cos(eulers3),-cos(eulers1).*sin(eulers3)+cos(eulers3).*sin(eulers1).*sin(eulers2),sin(eulers1).*sin(eulers3)+cos(eulers1).*cos(eulers3).*sin(eulers2),cos(eulers2).*sin(eulers3),cos(eulers1).*cos(eulers3)+sin(eulers1).*sin(eulers2).*sin(eulers3),-cos(eulers3).*sin(eulers1)+cos(eulers1).*sin(eulers2).*sin(eulers3),-sin(eulers2),cos(eulers2).*sin(eulers1),cos(eulers1).*cos(eulers2),0.0,r_dot_dot1.*(sin(eulers1).*sin(eulers3)+cos(eulers1).*cos(eulers3).*sin(eulers2))-r_dot_dot2.*(cos(eulers3).*sin(eulers1)-cos(eulers1).*sin(eulers2).*sin(eulers3))+r_dot_dot3.*cos(eulers1).*cos(eulers2),r_dot_dot1.*(cos(eulers1).*sin(eulers3)-cos(eulers3).*sin(eulers1).*sin(eulers2))-r_dot_dot2.*(cos(eulers1).*cos(eulers3)+sin(eulers1).*sin(eulers2).*sin(eulers3))-r_dot_dot3.*cos(eulers2).*sin(eulers1),-r_dot_dot3.*cos(eulers2)-r_dot_dot1.*cos(eulers3).*sin(eulers2)-r_dot_dot2.*sin(eulers2).*sin(eulers3),-r_dot_dot3.*sin(eulers1).*sin(eulers2)+r_dot_dot1.*cos(eulers2).*cos(eulers3).*sin(eulers1)+r_dot_dot2.*cos(eulers2).*sin(eulers1).*sin(eulers3),-r_dot_dot3.*cos(eulers1).*sin(eulers2)+r_dot_dot1.*cos(eulers1).*cos(eulers2).*cos(eulers3)+r_dot_dot2.*cos(eulers1).*cos(eulers2).*sin(eulers3),r_dot_dot2.*cos(eulers2).*cos(eulers3)-r_dot_dot1.*cos(eulers2).*sin(eulers3),-r_dot_dot1.*(cos(eulers1).*cos(eulers3)+sin(eulers1).*sin(eulers2).*sin(eulers3))-r_dot_dot2.*(cos(eulers1).*sin(eulers3)-cos(eulers3).*sin(eulers1).*sin(eulers2)),r_dot_dot1.*(cos(eulers3).*sin(eulers1)-cos(eulers1).*sin(eulers2).*sin(eulers3))+r_dot_dot2.*(sin(eulers1).*sin(eulers3)+cos(eulers1).*cos(eulers3).*sin(eulers2)),0.0,0.0,0.0,0.0,0.0,0.0,0.0,0.0,0.0,0.0,0.0,0.0,0.0,0.0,0.0,0.0,0.0,0.0,0.0,0.0,0.0,0.0,0.0,0.0,0.0,0.0,0.0],[3,21]);
H_jacobian_omega = [zeros(3,15),eye(3),zeros(3,3)];

prediction_full = [accel_prediction; omega_prediction; rho_prediction];
H_jacobian_full = [H_jacobian_accel; H_jacobian_omega; H_jacobian_rho];

if sum(sensor_vec) ~= 0
    sensor_indicies = sensor_vec==1;
    H = H_jacobian_full(sensor_indicies,:);
    R = R_full(sensor_indicies,sensor_indicies);
    prediction = prediction_full(sensor_indicies);
    z = z_full(sensor_indicies);
    
    y = z - prediction;
    S = H*P_hat_1*H' + R;
    K = P_hat_1*H'*inv(S);
    x_hat_2 = x_hat_1 + K*y;
    P_hat_2 = (eye(num_states) - K*H)*P_hat_1;
else
    x_hat_2 = x_hat_1;
    P_hat_2 = P_hat_1;
end

x_hat_2_prior = x_hat_2;
P_hat_2_prior = P_hat_2;

== matlab function EKF/Camera/MATLAB Function1 ==
  data: u input; y output
function y = fcn(u)

soft_max = exp(-u)./sum(exp(-u));

y = soft_max;
